simulink model "flyingcap5lvl"  (R2023b)
settings: Solver=ode4  StartTime=0.0  StopTime=0.1  FixedStep=1e-5  RelTol=1e-3  EnableMultiTasking=on
libraries: spsSeriesRLCBranchLib x12, spsVoltageMeasurementLib x9, spsIGBTDiodeLib x8, simulink x4, spsCurrentMeasurementLib x3, spsGroundLib x2, spsDCVoltageSourceLib x1, spspowerguiLib x1
settings Model: Creator=Ranit  LastModifiedBy=user
settings SolverCC: AlgebraicLoopSolver=TrustRegion
settings DataIOCC: ReturnWorkspaceOutputs=off
settings OptimizationCC: LifeSpan=inf
settings DebuggingCC: UnconnectedInputMsg=warning  UnconnectedOutputMsg=warning  UnconnectedLineMsg=warning  SFUnexpectedBacktrackingDiag=warning  SFNoUnconditionalDefaultTransitionDiag=warning  ArithmeticOperatorsInVariantConditions=warning
settings ModelReferenceCC: EnableRefExpFcnMdlSchedulingChecks=on
settings SFSimCC: SimUseLocalCustomCode=off  CustomCodeUndefinedFunction=UseInterfaceOnly
settings RTWCC: RTWUseLocalCustomCode=off
settings CodeAppCC: StateflowObjectComments=on
settings GRTTargetCC: TargetLangStandard=C89/C90 (ANSI)
settings ConfigComp: CovMetricSettings=dw  CovSaveCumulativeToWorkspaceVar=on  CovSaveSingleToWorkspaceVar=on  CovExternalEMLEnable=off
settings SimscapeCC: SimscapeNormalizeSystem=off

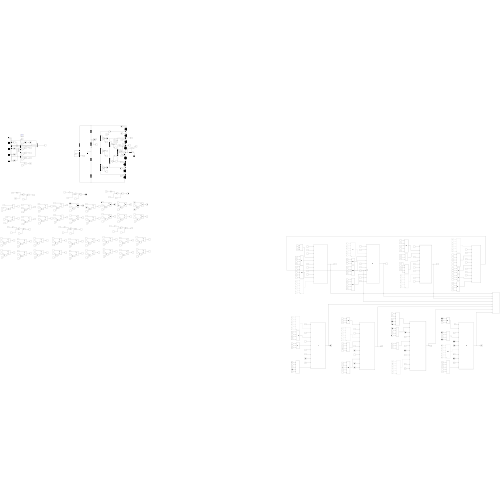
[thumbnail: Simulink's stored preview of the top-level diagram]
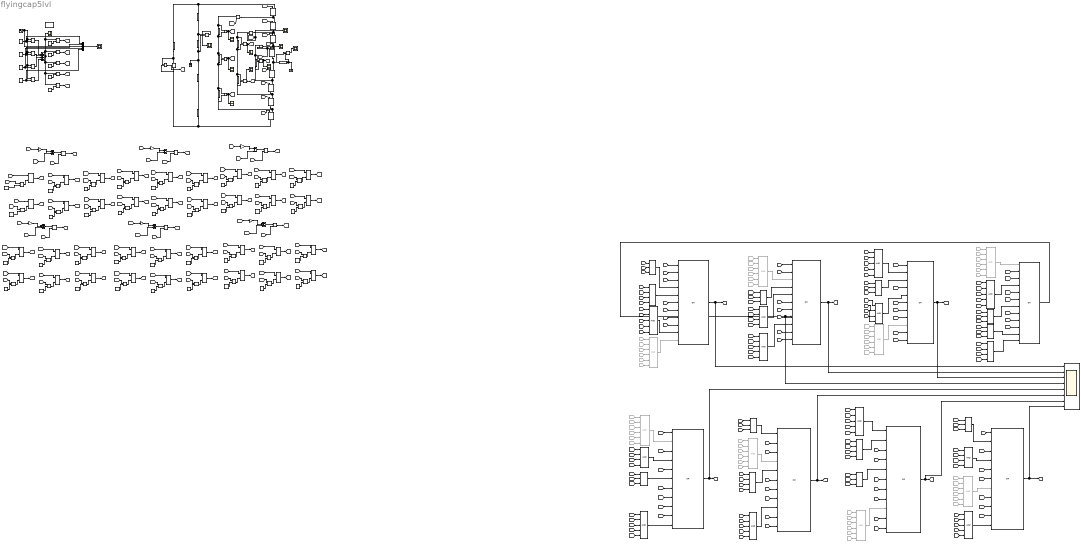
== system flyingcap5lvl ==
  Constant : Constant  Value=4
  Constant1 : Constant  Value=3
  Constant{4..40} (37 alike) : Constant  Value=0
  Constant2 : Constant  Value=2
  Constant3 : Constant
  Current Measurement1 : spsCurrentMeasurementLib/Current Measurement  PhasorSimulation=off  OutputType=Complex  PSBequivalent=0
  Current Measurement2 : spsCurrentMeasurementLib/Current Measurement  PhasorSimulation=off  OutputType=Complex  PSBequivalent=0
  Current Measurement3 : spsCurrentMeasurementLib/Current Measurement  PhasorSimulation=off  OutputType=Complex  PSBequivalent=0
  DC Voltage Source : spsDCVoltageSourceLib/DC Voltage Source  Amplitude=400  Measurements=None
  From{104,116,132,257} (4 alike) : From  Commented=on  GotoTag=c32
  From{113,135,206,258} (4 alike) : From  Commented=on  GotoTag=c42d
  From{34,121,129,279} (4 alike) : From  Commented=on  GotoTag=c32d
  From{98,122,194,280} (4 alike) : From  Commented=on  GotoTag=c42
  From{140,207,236,259} (4 alike) : From  Commented=on  GotoTag=c52d
  From{145,195,223,275} (4 alike) : From  Commented=on  GotoTag=c52
  From{196,224,244,276} (4 alike) : From  Commented=on  GotoTag=c62
  From{208,237,260,288} (4 alike) : From  Commented=on  GotoTag=c62d
  From{23,225,245,277} (4 alike) : From  Commented=on  GotoTag=c12
  From{91,226,246,278} (4 alike) : From  Commented=on  GotoTag=c22d
  From{95,238,261,289} (4 alike) : From  Commented=on  GotoTag=c12d
  From{96,239,262,290} (4 alike) : From  Commented=on  GotoTag=c22
  Gain{,1..5} (6 alike) : Gain  Gain=1/4
  Ground : spsGroundLib/Ground  LConnTagsString=a
  Ground1 : spsGroundLib/Ground  LConnTagsString=a
  IGBT/Diode{1..8} (8 alike) : spsIGBTDiodeLib/IGBT//Diode  Ron=1e-3  Rs=1e5  Cs=inf  Measurements=off
  Logical Operator{,1..5,14..25,42..59} (36 alike) : Logic  AllPortsSameDT=off  OutDataTypeStr=boolean
  Logical Operator{10..13,38..40} (7 alike) : Logic  Operator=OR  Inputs=11  AllPortsSameDT=off  OutDataTypeStr=boolean
  Logical Operator{26,36,61..62,68..69,72,75} (8 alike) : Logic  Inputs=4  AllPortsSameDT=off  OutDataTypeStr=boolean
  Logical Operator{6,8,27..29,31..32,35,37} (9 alike) : Logic  Inputs=3  AllPortsSameDT=off  OutDataTypeStr=boolean
  Logical Operator{7,9,30,34,65,67,71,74} (8 alike) : Logic  Commented=on  Inputs=6  AllPortsSameDT=off  OutDataTypeStr=boolean
  Logical Operator{33,60,63..64,66,70,73,76} (8 alike) : Logic  Inputs=5  AllPortsSameDT=off  OutDataTypeStr=boolean
  Logical Operator41 : Logic  Operator=OR  Inputs=12  AllPortsSameDT=off  OutDataTypeStr=boolean
  Mux : Mux  Inputs=5
  Product{,1..5} (6 alike) : Product
  Relational Operator{,1..3} (4 alike) : RelationalOperator  OutDataTypeStr=boolean  InputSameDT=off
  Relational Operator{10..11,13..15,18,21..22,24,27..28,30,33..34,36,39..40,42} (18 alike) : RelationalOperator  Operator=<  OutDataTypeStr=boolean  InputSameDT=off
  Relational Operator{9,12,16..17,19..20,23,25..26,29,31..32,35,37..38,41,43..44} (18 alike) : RelationalOperator  Operator=>  OutDataTypeStr=boolean  InputSameDT=off
  Relational Operator{4..8} (5 alike) : RelationalOperator  Operator===  OutDataTypeStr=boolean  InputSameDT=off
  Repeating Sequence : simulink/Sources/Repeating Sequence  rep_seq_t=[0 1 2]*[1/14000]  rep_seq_y=[0.5 1 0.5]
  Repeating Sequence1 : simulink/Sources/Repeating Sequence  rep_seq_t=[0 1 2]*[1/14000]  rep_seq_y=[0 0.5 0]
  Repeating Sequence2 : simulink/Sources/Repeating Sequence  rep_seq_t=[0 1 2]*[1/14000]  rep_seq_y=[-0.5 0 -0.5]
  Repeating Sequence3 : simulink/Sources/Repeating Sequence  rep_seq_t=[0 1 2]*[1/14000]  rep_seq_y=[-1 -0.5 -1]
  Scope{,1..11} (12 alike) : Scope
  Scope12 : Scope  NumInputPorts=8
  Series RLC Branch{,1..2,6..9} (7 alike) : spsSeriesRLCBranchLib/Series RLC Branch  LConnTagsString=__new0  RConnTagsString=__new0  BranchType=RC  Resistance=0.1  Inductance=1e-3  SetiL0=off  InitialCurrent=0  Capacitance=4.7e-3  Setx0=off  InitialVoltage=0  Measurements=None
  Series RLC Branch10 : spsSeriesRLCBranchLib/Series RLC Branch  LConnTagsString=__new0  RConnTagsString=__new0  BranchType=R  Resistance=50  Inductance=1e-3  SetiL0=off  InitialCurrent=0  Capacitance=4.7e-3  Setx0=off  InitialVoltage=0  Measurements=None
  Series RLC Branch11 : spsSeriesRLCBranchLib/Series RLC Branch  LConnTagsString=__new0  RConnTagsString=__new0  BranchType=R  Resistance=0.0001  Inductance=1e-4  SetiL0=off  InitialCurrent=0  Capacitance=4.7e-3  Setx0=off  InitialVoltage=0  Measurements=None
  Series RLC Branch3 : spsSeriesRLCBranchLib/Series RLC Branch  LConnTagsString=__new0  RConnTagsString=__new0  BranchType=RC  Resistance=0.034  Inductance=1e-3  SetiL0=off  InitialCurrent=0  Capacitance=4.7e-3  Setx0=off  InitialVoltage=0  Measurements=None
  Series RLC Branch4 : spsSeriesRLCBranchLib/Series RLC Branch  LConnTagsString=__new0  RConnTagsString=__new0  BranchType=RC  Resistance=0.034  Inductance=1e-3  SetiL0=off  InitialCurrent=0  Capacitance=4.7e-3  Setx0=off  InitialVoltage=0  Measurements=None
  Series RLC Branch5 : spsSeriesRLCBranchLib/Series RLC Branch  LConnTagsString=__new0  RConnTagsString=__new0  BranchType=RC  Resistance=0.034  Inductance=1e-3  SetiL0=off  InitialCurrent=0  Capacitance=4.7e-3  Setx0=off  InitialVoltage=0  Measurements=None
  Sine Wave : Sin  Frequency=2*pi*50  SampleTime=0
  Sum : Sum  Inputs=|++++
  Sum{1..6} (6 alike) : Sum  Inputs=|+-
  Vc{1..6} (6 alike) : spsVoltageMeasurementLib/Voltage Measurement  PhasorSimulation=off  OutputType=Complex  PSBequivalent=0
  Voltage Measurement1 : spsVoltageMeasurementLib/Voltage Measurement  PhasorSimulation=off  OutputType=Complex  PSBequivalent=0
  Voltage Measurement2 : spsVoltageMeasurementLib/Voltage Measurement  PhasorSimulation=off  OutputType=Complex  PSBequivalent=0
  Voltage Measurement3 : spsVoltageMeasurementLib/Voltage Measurement  PhasorSimulation=off  OutputType=Complex  PSBequivalent=0
  powergui : spspowerguiLib/powergui  Priority=1  SimulationMode=Discrete  SampleTime=1e-5  frequency=60  Iterations=50  frequencyindice=0  Pbase=100e6  ErrMax=1e-4  UnitsV=kV  UnitsW=MW  buscounter=0  FunctionMessages=off  echomessages=off  EnableUseOfTLC=off  CurrentSourceSwitches=off  DisableSnubberDevices=off  DisableRonSwitches=off  DisableVfSwitches=off  DisplayEquations=off  AutomaticDiscreteSolvers=off  SolverType=Tustin/Backward Euler (TBE)  Interpol=off  ExternalGateDelay=off  methode=off  Ts=10  x0status=blocks  SPID=off  SwTol=0  HookPort=off  NonlinearTolerance=1e-4  nMaxIteration=100  ContinueOnMaxIteration=off  RestoreLinks=warning  ResistiveCurrentMeasurement=off  Frange=[0:2:500]  Ylog=off  Xlog=on  ShowGrid=off  save=off  variable=ZData  structure=ScopeData1  ZoomFFT=off  StartTime=9.91  cycles=1  DisplayStyle=1  fundamental=50  FreqAxis=off  MaxFrequency=1000  frequencyindicesteady=1  RmsSteady=1  display=off
  wires:
  Sine Wave/1 -> Mux/3, Relational Operator/1, Relational Operator1/1, Relational Operator3/1, Relational Operator2/1
  Repeating Sequence/1 -> Mux/1, Relational Operator/2
  Repeating Sequence1/1 -> Mux/2, Relational Operator1/2
  Repeating Sequence2/1 -> Mux/4, Relational Operator2/2
  Repeating Sequence3/1 -> Mux/5, Relational Operator3/2
  Relational Operator/1 -> Sum/1
  Relational Operator1/1 -> Sum/2
  Relational Operator2/1 -> Sum/3
  Relational Operator3/1 -> Sum/4
  Sum/1 -> Relational Operator8/1, Relational Operator7/1, Relational Operator6/1, Scope3/1, Relational Operator4/1, Relational Operator5/1
  Relational Operator4/1 -> [pwm4]
  Relational Operator5/1 -> [pwm3]
  Relational Operator6/1 -> [pwm2]
  Relational Operator7/1 -> [pwm1]
  Relational Operator8/1 -> [pwm0]
  Constant4/1 -> Relational Operator8/2
  Constant3/1 -> Relational Operator7/2
  Constant2/1 -> Relational Operator6/2
  Constant1/1 -> Relational Operator5/2
  Constant/1 -> Relational Operator4/2
  Vc1/1 -> Scope4/1, [vc1]
  Voltage Measurement3/1 -> [Vdc]
  Voltage Measurement1/1 -> Scope1/1
  [s8] -> IGBT/Diode8/1
  [s7] -> IGBT/Diode7/1
  [s6] -> IGBT/Diode6/1
  [s5] -> IGBT/Diode5/1
  [s4] -> IGBT/Diode4/1
  [s3] -> IGBT/Diode3/1
  [s2] -> IGBT/Diode1/1
  [s1] -> IGBT/Diode2/1
  Voltage Measurement2/1 -> Scope2/1
  Current Measurement2/1 -> [ic1], Scope8/1
  [Vdc] -> Gain/1
  Gain/1 -> Sum1/1
  [vc1] -> Sum1/2
  Sum1/1 -> Product/1
  [ic1] -> Product/2
  Product/1 -> [sig1]
  Constant5/1 -> Relational Operator9/2
  [sig1] -> Relational Operator9/1
  [pwm3] -> Logical Operator1/1
  [sig1] -> Relational Operator12/1
  [pwm2] -> Logical Operator3/1
  Logical Operator2/1 -> [c12]
  [pwm2] -> Logical Operator2/1
  Logical Operator3/1 -> [c12d]
  [sig1] -> Relational Operator11/1
  Constant8/1 -> Relational Operator11/2
  Relational Operator12/1 -> Logical Operator2/2
  Constant7/1 -> Relational Operator12/2
  Relational Operator11/1 -> Logical Operator3/2
  Constant6/1 -> Relational Operator10/2
  [sig1] -> Relational Operator10/1
  [pwm3] -> Logical Operator/1
  [sig1] -> Relational Operator16/1
  Constant9/1 -> Relational Operator16/2
  [sig1] -> Relational Operator13/1
  Relational Operator13/1 -> Logical Operator5/2
  [pwm1] -> Logical Operator4/1
  Constant10/1 -> Relational Operator13/2
  [pwm1] -> Logical Operator5/1
  Relational Operator16/1 -> Logical Operator4/2
  Logical Operator5/1 -> [c11d]
  Logical Operator4/1 -> [c11]
  Relational Operator9/1 -> Logical Operator/2
  Relational Operator10/1 -> Logical Operator1/2
  Logical Operator1/1 -> [c13d]
  Logical Operator/1 -> [c13]
  Vc2/1 -> Scope5/1, [vc2]
  Vc3/1 -> Scope6/1, [vc3]
  [Vdc] -> Gain1/1
  Gain1/1 -> Sum2/1
  [vc2] -> Sum2/2
  Sum2/1 -> Product1/1
  Product1/1 -> [sig2]
  [Vdc] -> Gain2/1
  Gain2/1 -> Sum3/1
  [vc3] -> Sum3/2
  Sum3/1 -> Product2/1
  Product2/1 -> [sig3]
  Constant12/1 -> Relational Operator20/2
  [sig2] -> Relational Operator20/1
  [pwm3] -> Logical Operator15/1
  [sig2] -> Relational Operator17/1
  [pwm2] -> Logical Operator17/1
  Logical Operator16/1 -> [c22]
  [pwm2] -> Logical Operator16/1
  Logical Operator17/1 -> [c22d]
  [sig2] -> Relational Operator15/1
  Constant15/1 -> Relational Operator15/2
  Relational Operator17/1 -> Logical Operator16/2
  Constant14/1 -> Relational Operator17/2
  Relational Operator15/1 -> Logical Operator17/2
  Constant13/1 -> Relational Operator14/2
  [sig2] -> Relational Operator14/1
  [pwm3] -> Logical Operator14/1
  [sig2] -> Relational Operator19/1
  Constant16/1 -> Relational Operator19/2
  [sig2] -> Relational Operator18/1
  Relational Operator18/1 -> Logical Operator19/2
  [pwm1] -> Logical Operator18/1
  Constant11/1 -> Relational Operator18/2
  [pwm1] -> Logical Operator19/1
  Relational Operator19/1 -> Logical Operator18/2
  Logical Operator19/1 -> [c21d]
  Logical Operator18/1 -> [c21]
  Relational Operator20/1 -> Logical Operator14/2
  Relational Operator14/1 -> Logical Operator15/2
  Logical Operator15/1 -> [c23d]
  Logical Operator14/1 -> [c23]
  Constant18/1 -> Relational Operator26/2
  [sig3] -> Relational Operator26/1
  [pwm3] -> Logical Operator21/1
  [sig3] -> Relational Operator23/1
  [pwm2] -> Logical Operator23/1
  Logical Operator22/1 -> [c32]
  [pwm2] -> Logical Operator22/1
  Logical Operator23/1 -> [c32d]
  [sig3] -> Relational Operator22/1
  Constant21/1 -> Relational Operator22/2
  Relational Operator23/1 -> Logical Operator22/2
  Constant20/1 -> Relational Operator23/2
  Relational Operator22/1 -> Logical Operator23/2
  Constant19/1 -> Relational Operator21/2
  [sig3] -> Relational Operator21/1
  [pwm3] -> Logical Operator20/1
  [sig3] -> Relational Operator25/1
  Constant22/1 -> Relational Operator25/2
  [sig3] -> Relational Operator24/1
  Relational Operator24/1 -> Logical Operator25/2
  [pwm1] -> Logical Operator24/1
  Constant17/1 -> Relational Operator24/2
  [pwm1] -> Logical Operator25/1
  Relational Operator25/1 -> Logical Operator24/2
  Logical Operator25/1 -> [c31d]
  Logical Operator24/1 -> [c31]
  Relational Operator26/1 -> Logical Operator20/2
  Relational Operator21/1 -> Logical Operator21/2
  Logical Operator21/1 -> [c33d]
  Logical Operator20/1 -> [c33]
  Current Measurement1/1 -> Scope7/1, [ic23]
  [ic23] -> Product1/2
  [ic23] -> Product2/2
  [c13] -> Logical Operator38/1
  [pwm4] -> Logical Operator38/3
  Logical Operator38/1 -> Scope12/1, [s1]
  [c13] -> Logical Operator39/1
  Logical Operator39/1 -> Scope12/2, [s2]
  [c13] -> Logical Operator40/1
  [c13] -> Logical Operator10/1
  Logical Operator32/1 -> Logical Operator11/1
  [c11d] -> Logical Operator11/3
  [c11d] -> Logical Operator12/3
  [pwm0] -> Logical Operator12/4
  [c11d] -> Logical Operator13/3
  Logical Operator13/1 -> Scope12/8, [s8]
  [c23] -> Logical Operator6/2
  [c13d] -> Logical Operator6/1
  Logical Operator6/1 -> Logical Operator38/4
  From23/1 -> Logical Operator7/1
  From91/1 -> Logical Operator7/2
  [c23] -> Logical Operator8/2
  [c13d] -> Logical Operator8/1
  From96/1 -> Logical Operator9/2
  From95/1 -> Logical Operator9/1
  [c21d] -> Logical Operator27/2
  [c11] -> Logical Operator27/1
  Logical Operator27/1 -> Logical Operator40/3
  [c23] -> Logical Operator28/2
  [c13d] -> Logical Operator28/1
  [c22] -> Logical Operator29/2
  [c12d] -> Logical Operator29/1
  [c21d] -> Logical Operator31/2
  [c11] -> Logical Operator31/1
  [c23] -> Logical Operator32/2
  [c13d] -> Logical Operator32/1
  [c21d] -> Logical Operator35/2
  [c11] -> Logical Operator35/1
  [c21d] -> Logical Operator37/2
  [c11] -> Logical Operator37/1
  [c22] -> Logical Operator38/2
  Logical Operator37/1 -> Logical Operator13/2
  [c33] -> Logical Operator6/3
  From129/1 -> Logical Operator7/3
  From132/1 -> Logical Operator9/3
  [c33] -> Logical Operator8/3
  [c31d] -> Logical Operator27/3
  [c33] -> Logical Operator28/3
  [c11d] -> Logical Operator41/2
  [pwm4] -> Logical Operator41/3
  [c32] -> Logical Operator29/3
  [c31d] -> Logical Operator37/3
  [c31d] -> Logical Operator35/3
  [c33] -> Logical Operator32/3
  [pwm0] -> Logical Operator11/2
  [c31d] -> Logical Operator31/3
  [pwm0] -> Logical Operator10/3
  Logical Operator31/1 -> Logical Operator10/6
  [Vdc] -> Gain3/1
  Gain3/1 -> Sum4/1
  [vc5] -> Sum4/2
  Sum4/1 -> Product3/1
  Product3/1 -> [sig5]
  Constant24/1 -> Relational Operator32/2
  [sig5] -> Relational Operator32/1
  [pwm3] -> Logical Operator43/1
  [sig5] -> Relational Operator29/1
  [pwm2] -> Logical Operator45/1
  Logical Operator44/1 -> [c52]
  [pwm2] -> Logical Operator44/1
  Logical Operator45/1 -> [c52d]
  [sig5] -> Relational Operator28/1
  Constant27/1 -> Relational Operator28/2
  Relational Operator29/1 -> Logical Operator44/2
  Constant26/1 -> Relational Operator29/2
  Relational Operator28/1 -> Logical Operator45/2
  Constant25/1 -> Relational Operator27/2
  [sig5] -> Relational Operator27/1
  [pwm3] -> Logical Operator42/1
  [sig5] -> Relational Operator31/1
  Constant28/1 -> Relational Operator31/2
  [sig5] -> Relational Operator30/1
  Relational Operator30/1 -> Logical Operator47/2
  [pwm1] -> Logical Operator46/1
  Constant23/1 -> Relational Operator30/2
  [pwm1] -> Logical Operator47/1
  Relational Operator31/1 -> Logical Operator46/2
  Logical Operator47/1 -> [c51d]
  Logical Operator46/1 -> [c51]
  Relational Operator32/1 -> Logical Operator42/2
  Relational Operator27/1 -> Logical Operator43/2
  Logical Operator43/1 -> [c53d]
  Logical Operator42/1 -> [c53]
  [ic456] -> Product3/2
  [Vdc] -> Gain4/1
  Gain4/1 -> Sum5/1
  [vc4] -> Sum5/2
  Sum5/1 -> Product4/1
  Product4/1 -> [sig4]
  Constant30/1 -> Relational Operator38/2
  [sig4] -> Relational Operator38/1
  [pwm3] -> Logical Operator49/1
  [sig4] -> Relational Operator35/1
  [pwm2] -> Logical Operator51/1
  Logical Operator50/1 -> [c42]
  [pwm2] -> Logical Operator50/1
  Logical Operator51/1 -> [c42d]
  [sig4] -> Relational Operator34/1
  Constant33/1 -> Relational Operator34/2
  Relational Operator35/1 -> Logical Operator50/2
  Constant32/1 -> Relational Operator35/2
  Relational Operator34/1 -> Logical Operator51/2
  Constant31/1 -> Relational Operator33/2
  [sig4] -> Relational Operator33/1
  [pwm3] -> Logical Operator48/1
  [sig4] -> Relational Operator37/1
  Constant34/1 -> Relational Operator37/2
  [sig4] -> Relational Operator36/1
  Relational Operator36/1 -> Logical Operator53/2
  [pwm1] -> Logical Operator52/1
  Constant29/1 -> Relational Operator36/2
  [pwm1] -> Logical Operator53/1
  Relational Operator37/1 -> Logical Operator52/2
  Logical Operator53/1 -> [c41d]
  Logical Operator52/1 -> [c41]
  Relational Operator38/1 -> Logical Operator48/2
  Relational Operator33/1 -> Logical Operator49/2
  Logical Operator49/1 -> [c43d]
  Logical Operator48/1 -> [c43]
  [ic456] -> Product4/2
  [Vdc] -> Gain5/1
  Gain5/1 -> Sum6/1
  [vc6] -> Sum6/2
  Sum6/1 -> Product5/1
  Product5/1 -> [sig6]
  Constant36/1 -> Relational Operator44/2
  [sig6] -> Relational Operator44/1
  [pwm3] -> Logical Operator55/1
  [sig6] -> Relational Operator41/1
  [pwm2] -> Logical Operator57/1
  Logical Operator56/1 -> [c62]
  [pwm2] -> Logical Operator56/1
  Logical Operator57/1 -> [c62d]
  [sig6] -> Relational Operator40/1
  Constant39/1 -> Relational Operator40/2
  Relational Operator41/1 -> Logical Operator56/2
  Constant38/1 -> Relational Operator41/2
  Relational Operator40/1 -> Logical Operator57/2
  Constant37/1 -> Relational Operator39/2
  [sig6] -> Relational Operator39/1
  [pwm3] -> Logical Operator54/1
  [sig6] -> Relational Operator43/1
  Constant40/1 -> Relational Operator43/2
  [sig6] -> Relational Operator42/1
  Relational Operator42/1 -> Logical Operator59/2
  [pwm1] -> Logical Operator58/1
  Constant35/1 -> Relational Operator42/2
  [pwm1] -> Logical Operator59/1
  Relational Operator43/1 -> Logical Operator58/2
  Logical Operator59/1 -> [c61d]
  Logical Operator58/1 -> [c61]
  Relational Operator44/1 -> Logical Operator54/2
  Relational Operator39/1 -> Logical Operator55/2
  Logical Operator55/1 -> [c63d]
  Logical Operator54/1 -> [c63]
  [ic456] -> Product5/2
  Current Measurement3/1 -> [ic456]
  Vc4/1 -> Scope9/1, [vc4]
  Vc5/1 -> Scope10/1, [vc5]
  Vc6/1 -> Scope11/1, [vc6]
  [c43] -> Logical Operator60/1
  [c53] -> Logical Operator60/2
  [c63] -> Logical Operator60/3
  [c33d] -> Logical Operator60/4
  [c23d] -> Logical Operator60/5
  From194/1 -> Logical Operator7/4
  From195/1 -> Logical Operator7/5
  From196/1 -> Logical Operator7/6
  [c12d] -> Logical Operator61/1
  [c42] -> Logical Operator61/2
  [c52] -> Logical Operator61/3
  [c62] -> Logical Operator61/4
  Logical Operator7/1 -> Logical Operator38/11
  Logical Operator60/1 -> Logical Operator38/10
  [c32] -> Logical Operator38/6
  [c41] -> Logical Operator38/7
  [c51] -> Logical Operator38/8
  [c61] -> Logical Operator38/9
  From206/1 -> Logical Operator9/4
  From207/1 -> Logical Operator9/5
  From208/1 -> Logical Operator9/6
  [c42d] -> Logical Operator62/1
  [c52d] -> Logical Operator62/2
  [c62d] -> Logical Operator62/3
  [c12] -> Logical Operator62/4
  [c21] -> Logical Operator63/1
  [c31] -> Logical Operator63/2
  [c41d] -> Logical Operator63/3
  [c51d] -> Logical Operator63/4
  [c61d] -> Logical Operator63/5
  [pwm4] -> Logical Operator39/2
  Logical Operator9/1 -> Logical Operator39/3
  Logical Operator8/1 -> Logical Operator39/4
  Logical Operator62/1 -> Logical Operator39/5
  [c43d] -> Logical Operator39/6
  [c53d] -> Logical Operator39/7
  [c63d] -> Logical Operator39/8
  Logical Operator63/1 -> Logical Operator39/9
  [c43] -> Logical Operator64/1
  [c53] -> Logical Operator64/2
  [c63] -> Logical Operator64/3
  [c33d] -> Logical Operator64/4
  [c23d] -> Logical Operator64/5
  From225/1 -> Logical Operator65/1
  From226/1 -> Logical Operator65/2
  From34/1 -> Logical Operator65/3
  From98/1 -> Logical Operator65/4
  From223/1 -> Logical Operator65/5
  From224/1 -> Logical Operator65/6
  [c42d] -> Logical Operator26/1
  [c52d] -> Logical Operator26/2
  [c62d] -> Logical Operator26/3
  [c12] -> Logical Operator26/4
  Logical Operator64/1 -> Logical Operator40/2
  [pwm4] -> Logical Operator40/4
  Logical Operator26/1 -> Logical Operator40/5
  [c53d] -> Logical Operator40/7
  [c43d] -> Logical Operator40/6
  [c63d] -> Logical Operator40/8
  Logical Operator65/1 -> Logical Operator40/9
  [c43] -> Logical Operator66/1
  [c53] -> Logical Operator66/2
  [c63] -> Logical Operator66/3
  [c33d] -> Logical Operator66/4
  [c23d] -> Logical Operator66/5
  From239/1 -> Logical Operator67/2
  From238/1 -> Logical Operator67/1
  From116/1 -> Logical Operator67/3
  From135/1 -> Logical Operator67/4
  From236/1 -> Logical Operator67/5
  From237/1 -> Logical Operator67/6
  [c12d] -> Logical Operator68/1
  [c42] -> Logical Operator68/2
  [c52] -> Logical Operator68/3
  [c62] -> Logical Operator68/4
  Logical Operator67/1 -> Logical Operator41/1
  Logical Operator66/1 -> Logical Operator41/4
  [c22d] -> Logical Operator41/5
  [c32d] -> Logical Operator41/6
  Logical Operator29/1 -> Logical Operator41/7
  Logical Operator68/1 -> Logical Operator41/12
  Logical Operator28/1 -> Logical Operator41/11
  [c43d] -> Logical Operator41/8
  [c53d] -> Logical Operator41/9
  [c63d] -> Logical Operator41/10
  From245/1 -> Logical Operator30/1
  From246/1 -> Logical Operator30/2
  From121/1 -> Logical Operator30/3
  From122/1 -> Logical Operator30/4
  From145/1 -> Logical Operator30/5
  From244/1 -> Logical Operator30/6
  [c42d] -> Logical Operator69/1
  [c52d] -> Logical Operator69/2
  [c62d] -> Logical Operator69/3
  [c12] -> Logical Operator69/4
  [c21] -> Logical Operator70/1
  [c31] -> Logical Operator70/2
  [c41d] -> Logical Operator70/3
  [c51d] -> Logical Operator70/4
  [c61d] -> Logical Operator70/5
  Logical Operator30/1 -> Logical Operator10/2
  Logical Operator69/1 -> Logical Operator10/4
  [c32] -> Logical Operator10/5
  [c22] -> Logical Operator10/7
  [c41] -> Logical Operator10/8
  [c51] -> Logical Operator10/9
  [c61] -> Logical Operator10/10
  Logical Operator70/1 -> Logical Operator10/11
  From262/1 -> Logical Operator71/2
  From261/1 -> Logical Operator71/1
  From257/1 -> Logical Operator71/3
  From258/1 -> Logical Operator71/4
  From259/1 -> Logical Operator71/5
  From260/1 -> Logical Operator71/6
  [c12d] -> Logical Operator72/1
  [c42] -> Logical Operator72/2
  [c52] -> Logical Operator72/3
  [c62] -> Logical Operator72/4
  [c21] -> Logical Operator73/1
  [c31] -> Logical Operator73/2
  [c41d] -> Logical Operator73/3
  [c51d] -> Logical Operator73/4
  [c61d] -> Logical Operator73/5
  Logical Operator71/1 -> Logical Operator11/4
  [c41] -> Logical Operator11/6
  [c51] -> Logical Operator11/7
  [c61] -> Logical Operator11/8
  [c43] -> Logical Operator33/1
  [c53] -> Logical Operator33/2
  [c63] -> Logical Operator33/3
  [c33d] -> Logical Operator33/4
  [c23d] -> Logical Operator33/5
  From277/1 -> Logical Operator74/1
  From278/1 -> Logical Operator74/2
  From279/1 -> Logical Operator74/3
  From280/1 -> Logical Operator74/4
  From275/1 -> Logical Operator74/5
  From276/1 -> Logical Operator74/6
  [c12d] -> Logical Operator75/1
  [c42] -> Logical Operator75/2
  [c52] -> Logical Operator75/3
  [c62] -> Logical Operator75/4
  Logical Operator75/1 -> Logical Operator12/2
  Logical Operator33/1 -> Logical Operator12/1
  Logical Operator35/1 -> Logical Operator12/5
  [c41] -> Logical Operator12/6
  [c51] -> Logical Operator12/7
  [c61] -> Logical Operator12/8
  Logical Operator74/1 -> Logical Operator12/9
  From290/1 -> Logical Operator34/2
  From289/1 -> Logical Operator34/1
  From104/1 -> Logical Operator34/3
  From113/1 -> Logical Operator34/4
  From140/1 -> Logical Operator34/5
  From288/1 -> Logical Operator34/6
  [c42d] -> Logical Operator36/1
  [c52d] -> Logical Operator36/2
  [c62d] -> Logical Operator36/3
  [c12] -> Logical Operator36/4
  Logical Operator73/1 -> Logical Operator11/9
  [c21] -> Logical Operator76/1
  [c31] -> Logical Operator76/2
  [c41d] -> Logical Operator76/3
  [c51d] -> Logical Operator76/4
  [c61d] -> Logical Operator76/5
  [pwm0] -> Logical Operator13/1
  Logical Operator36/1 -> Logical Operator13/4
  [c22d] -> Logical Operator13/5
  [c32d] -> Logical Operator13/6
  Logical Operator34/1 -> Logical Operator13/7
  [c43d] -> Logical Operator13/8
  [c53d] -> Logical Operator13/9
  [c63d] -> Logical Operator13/10
  Logical Operator76/1 -> Logical Operator13/11
  [c22] -> Logical Operator11/10
  [c32] -> Logical Operator11/11
  [c22d] -> Logical Operator40/10
  [c32d] -> Logical Operator40/11
  Logical Operator61/1 -> Logical Operator38/5
  [c22] -> Logical Operator39/10
  [c32] -> Logical Operator39/11
  [c22d] -> Logical Operator12/10
  [c32d] -> Logical Operator12/11
  Logical Operator72/1 -> Logical Operator11/5
  Mux/1 -> Scope/1
  Logical Operator12/1 -> Scope12/7, [s7]
  Logical Operator11/1 -> Scope12/6, [s6]
  Logical Operator10/1 -> Scope12/5, [s5]
  Logical Operator40/1 -> Scope12/3, [s3]
  Logical Operator41/1 -> Scope12/4, [s4]
  connections:
  IGBT/Diode1/LConn1 -- Current Measurement3/LConn1 -- IGBT/Diode2/RConn1
  Current Measurement1/LConn1 -- IGBT/Diode1/RConn1 -- IGBT/Diode3/LConn1
  IGBT/Diode3/RConn1 -- Current Measurement2/LConn1 -- IGBT/Diode4/LConn1
  IGBT/Diode4/RConn1 -- Voltage Measurement1/LConn1 -- Series RLC Branch10/RConn1 -- IGBT/Diode5/LConn1
  IGBT/Diode5/RConn1 -- Vc1/LConn2 -- Series RLC Branch/RConn1 -- IGBT/Diode6/LConn1
  IGBT/Diode6/RConn1 -- Series RLC Branch2/RConn1 -- Vc3/LConn2 -- IGBT/Diode7/LConn1
  IGBT/Diode7/RConn1 -- Vc6/LConn2 -- Series RLC Branch5/RConn1 -- IGBT/Diode8/LConn1
  Series RLC Branch4/RConn1 -- Vc6/LConn1 -- Series RLC Branch5/LConn1 -- Vc5/LConn2
  DC Voltage Source/RConn1 -- Series RLC Branch11/RConn1 -- Voltage Measurement3/LConn1
  Series RLC Branch7/LConn1 -- Voltage Measurement2/LConn1 -- Series RLC Branch6/RConn1
  Series RLC Branch8/LConn1 -- Ground/LConn1 -- Voltage Measurement2/LConn2 -- Series RLC Branch7/RConn1
  Series RLC Branch9/LConn1 -- Series RLC Branch8/RConn1
  Series RLC Branch9/RConn1 -- Voltage Measurement3/LConn2 -- DC Voltage Source/LConn1 -- IGBT/Diode8/RConn1
  Series RLC Branch10/LConn1 -- Voltage Measurement1/LConn2 -- Ground1/LConn1
  Series RLC Branch3/RConn1 -- Vc5/LConn1 -- Series RLC Branch4/LConn1 -- Vc4/LConn2
  Current Measurement2/RConn1 -- Vc1/LConn1 -- Series RLC Branch/LConn1
  Current Measurement1/RConn1 -- Vc2/LConn1 -- Series RLC Branch1/LConn1
  Vc3/LConn1 -- Series RLC Branch2/LConn1 -- Vc2/LConn2 -- Series RLC Branch1/RConn1
  Series RLC Branch3/LConn1 -- Vc4/LConn1 -- Current Measurement3/RConn1
  Series RLC Branch6/LConn1 -- Series RLC Branch11/LConn1 -- IGBT/Diode2/LConn1
